simulink model "PathFollowing"  (R2018a)
settings: Solver=VariableStepAuto  StartTime=0.0  StopTime=10.0  RelTol=1e-3
undefined symbols (not defined in the file): SkywalkerX8
settings Model: Creator=David  LastModifiedBy=David

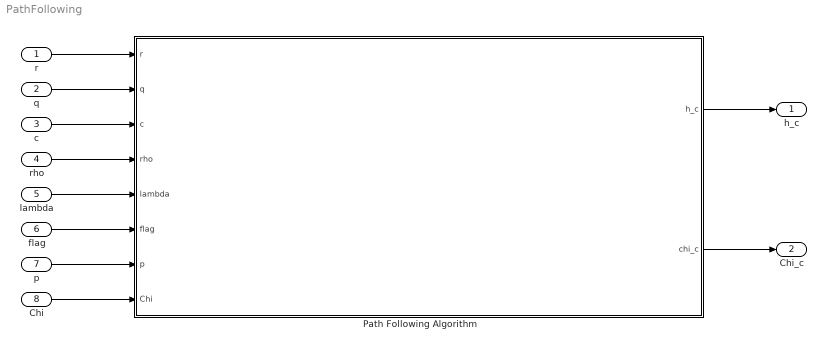
== system PathFollowing ==
  r : Inport
  q : Inport  Port=2
  c : Inport  Port=3
  rho : Inport  Port=4
  lambda : Inport  Port=5
  flag : Inport  Port=6
  p : Inport  Port=7
  Chi : Inport  Port=8
  Path Following Algorithm : Subsystem  mask{SampleTime=SkywalkerX8.GuidanceAndNavigation.SampleTime, ChiInf=SkywalkerX8.GuidanceAndNavigation.StraightLineFollowing.ChiInf, kpath=SkywalkerX8.GuidanceAndNavigation.StraightLineFollowing.kPath, korbit=SkywalkerX8.GuidanceAndNavigation.OrbitFollowing.kOrbit}
      mask prompts: SampleTime "Sample time (s)"; ChiInf "Chi_inf (rad)"; kpath "kPath (Unitless)"; korbit "kOrbit (Unitless)"
      mask DialogControl DescGroupVar Prompt: Path Following Algorithm
      mask DialogControl DescTextVar Prompt: The path following algorithms are implemented here with a straight line tracking and orbit following system being implemented. Which of these is active is dependant on the flag input.
      mask DialogControl Control2 Prompt: Flag = 1: Straight line following
      mask DialogControl Control3 Prompt: Flag = 2: Orbit following
      mask DialogControl Container4 Prompt: Straight Line Following
      mask DialogControl Control4 Prompt: Course angle when infinitely far from the path (rad)
      mask DialogControl Control5 Prompt: Course angle transition rate (how quickly we transition from Chi_Inf to Chi_d) (0 -> 1)
      mask DialogControl Container5 Prompt: Orbit Following
      mask DialogControl Control7 Prompt: Scalar for quickly we transition from moving toward the center of an orbit (the path we take when infinitely far from c) and to the ideal course angle command based on the orbit (ie. the course angle needed to maintain the orbit radius from the center)
      mask Display:
      | image('path_following.jpg')
      | 
      | port_label('input', 1, '\bf{r} (m)', 'texMode', 'On')
      | port_label('input', 2, '\bf{q} (m)', 'texMode', 'On')
      | port_label('input', 3, '\bf{c} (m)', 'texMode', 'On')
      | port_label('input', 4, '\rho (m)', 'texMode', 'On')
      | port_label('input', 5, '\lambda (Unitless)', 'texMode', 'On')
      | port_label('input', 6, 'Flag (Unitless)', 'texMode', 'On')
      | port_label('input', 7, '\bf{p} (m)', 'texMode', 'On')
      | port_label('input', 8, '\chi (rad)', 'texMode', 'On')
      | 
      | port_label('output', 1, 'h_c (m)', 'texMode', 'On')
      | port_label('output', 2, '\chi_c (rad)', 'texMode', 'On')
  h_c : Outport
  Chi_c : Outport  Port=2
  wires:
  r/1 -> Path Following Algorithm/1(r)
  q/1 -> Path Following Algorithm/2(q)
  c/1 -> Path Following Algorithm/3(c)
  rho/1 -> Path Following Algorithm/4(rho)
  p/1 -> Path Following Algorithm/7(p)
  Chi/1 -> Path Following Algorithm/8(Chi)
  Path Following Algorithm/1(h_c) -> h_c/1
  lambda/1 -> Path Following Algorithm/5(lambda)
  flag/1 -> Path Following Algorithm/6(flag)
  Path Following Algorithm/2(chi_c) -> Chi_c/1

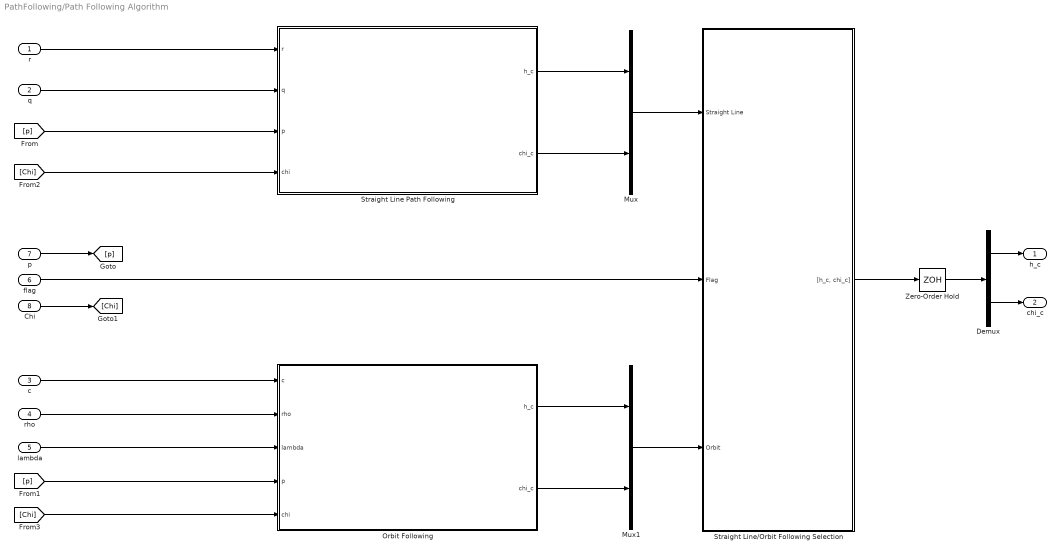
== system PathFollowing/Path Following Algorithm ==
  r : Inport
  q : Inport  Port=2
  c : Inport  Port=3
  rho : Inport  Port=4
  lambda : Inport  Port=5
  flag : Inport  Port=6
  p : Inport  Port=7
  Chi : Inport  Port=8
  Demux : Demux  Outputs=2
  Mux : Mux  Inputs=2
  Mux1 : Mux  Inputs=2
  Orbit Following : MATLAB Function  TreatAsAtomicUnit=on  mask{korbit=korbit}
      mask prompts: korbit "kOrbit (Unitless)"
  Straight Line Path Following : MATLAB Function  TreatAsAtomicUnit=on  mask{chi_inf=ChiInf, kpath=kpath}
      mask prompts: chi_inf "Chi_inf (rad)"; kpath "kPath (Unitless)"
  Straight Line/Orbit Following Selection : Subsystem
      mask Display:
      | port_label('input', 1, '[h_c, \chi_c]_{Straight Line} (m, rad)', 'texMode', 'On')
      | port_label('input', 2, 'Flag (Unitless)', 'texMode', 'On')
      | port_label('input', 3, '[h_c, \chi_c]_{Orbit Following} (m, rad)', 'texMode', 'On')
      | 
      | port_label('output', 1, '[h_c, \chi_c] (m, rad)', 'texMode', 'On')
  Zero-Order Hold : ZeroOrderHold  SampleTime=SampleTime
  h_c : Outport
  chi_c : Outport  Port=2
  wires:
  [Chi] -> Orbit Following/5(chi)
  rho/1 -> Orbit Following/2(rho)
  r/1 -> Straight Line Path Following/1(r)
  Orbit Following/2(chi_c) -> Mux1/2
  q/1 -> Straight Line Path Following/2(q)
  p/1 -> [p]
  lambda/1 -> Orbit Following/3(lambda)
  Orbit Following/1(h_c) -> Mux1/1
  Straight Line/Orbit Following Selection/1("[h_c, chi_c]") -> Zero-Order Hold/1
  Mux/1 -> Straight Line/Orbit Following Selection/1(Straight Line)
  c/1 -> Orbit Following/1(c)
  Mux1/1 -> Straight Line/Orbit Following Selection/3(Orbit)
  Straight Line Path Following/2(chi_c) -> Mux/2
  [Chi] -> Straight Line Path Following/4(chi)
  flag/1 -> Straight Line/Orbit Following Selection/2(Flag)
  [p] -> Straight Line Path Following/3(p)
  Straight Line Path Following/1(h_c) -> Mux/1
  Chi/1 -> [Chi]
  [p] -> Orbit Following/4(p)
  Zero-Order Hold/1 -> Demux/1
  Demux/1 -> h_c/1
  Demux/2 -> chi_c/1

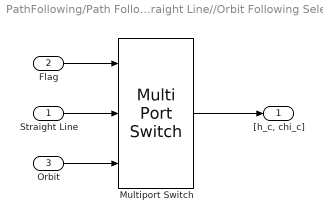
== system PathFollowing/Path Following Algorithm/Straight Line//Orbit Following Selection ==
  Straight Line : Inport
  Flag : Inport  Port=2
  Orbit : Inport  Port=3
  Multiport Switch : MultiPortSwitch  Inputs=2  DiagnosticForDefault=Warning
  "[h_c, chi_c]" : Outport
  wires:
  Orbit/1 -> Multiport Switch/3
  Flag/1 -> Multiport Switch/1
  Straight Line/1 -> Multiport Switch/2
  Multiport Switch/1 -> "[h_c, chi_c]"/1

== matlab function PathFollowing/Path Following Algorithm/Orbit Following ==
  data: c input size=3, 1; h_c output; rho input; lambda input; p input size=3, 1; chi input; chi_c output; korbit parameter
function [h_c, chi_c] = fcn(c, rho, lambda, p, chi, korbit)

    [h_c, chi_c] = orbitFollowing(c, rho, lambda, p, chi, korbit);

end

== matlab function PathFollowing/Path Following Algorithm/Straight Line Path Following ==
  data: r input size=3, 1; h_c output; chi_c output; q input size=3, 1; p input size=3, 1; chi input size=1; chi_inf parameter; kpath parameter
function [h_c, chi_c] = fcn(r, q, p, chi, chi_inf, kpath)

    [h_c, chi_c] = straightLineFollowing(r, q, p, chi, chi_inf, kpath);

end
